simulink model "COVID_mod"  (Simulink 10.1)
settings: Solver=ode4  StartTime=0.0  StopTime=400  FixedStep=1  MaxStep=1e-2  RelTol=1e-3
values from neighbouring files (symbols this model uses):
  alpha = 1 / str2double( get( handles.tau_inc, 'String' ) )    [covid.m]
  beta = R * (gamma + Delta)    [covid.m]
  D_init = 0    [covid.m]
  delta = gamma    [covid.m]
  dOldRate = get( handles.ElderlyDeath, 'Value' )    [covid.m]
  dRate = 1 - get( handles.Recover, 'Value' )    [covid.m]
  E_init = 20 * I_init    [covid.m]
  gamma = 1/str2double( get( handles.tau_rec, 'String' ) )    [covid.m]
  Hi = 1 + tol    (= 1.05)    [covid.m]
  I_init = n    [covid.m]
  Lo = 1 - tol    (= 0.95)    [covid.m]
  N = str2double( get( handles.N, 'String' ) )    [covid.m]
  oldPop = get( handles.Elderly, 'Value' )    [covid.m]
  otherPop = 1 - oldPop    [covid.m]
  R_init = 0    [covid.m]
  S_init = N - I_init - E_init - D_init - R_init    [covid.m]
  sigma = get( hObject, 'Value' )    [covid.m]
  tau_sigmapost = str2double( get( handles.tau_sigmapost, 'String' ) )    [covid.m]
  tau_sigmapre = str2double( get( handles.tau_sigmapre, 'String' ) )    [covid.m]
  tau_xi = str2double( get( handles.tau_xi, 'String' ) )    [covid.m]
  xi = get( handles.Resusceptible, 'Value' ) / 100    [covid.m]
libraries: simulink x3
settings Model: Creator=markng  LastModifiedBy=markng
settings DataIOCC: SaveFormat=Dataset  ReturnWorkspaceOutputs=on  OutputSaveName=out
settings DebuggingCC: AlgebraicLoopMsg=none  ArtificialAlgebraicLoopMsg=none  UnderspecifiedInitializationDetection=Simplified  MergeDetectMultiDrivingBlocksExec=error  SFUnexpectedBacktrackingDiag=error  SFNoUnconditionalDefaultTransitionDiag=error
settings HardwareCC: ProdBitPerPointer=64  ProdLargestAtomicFloat=Float  ProdIntDivRoundTo=Zero  ProdEndianess=LittleEndian  ProdHWDeviceType=Specified
settings ModelReferenceCC: PropagateSignalLabelsOutOfModel=on
settings SFSimCC: SimUseLocalCustomCode=on
settings RTWCC: RTWUseLocalCustomCode=on
settings GRTTargetCC: TargetLangStandard=C99 (ISO)  CombineOutputUpdateFcns=on  GRTInterface=off
settings ConfigComp: CovMetricSettings=dwe  CovHtmlReporting=off  CovSaveCumulativeToWorkspaceVar=off  CovSaveSingleToWorkspaceVar=off  CovExternalEMLEnable=on

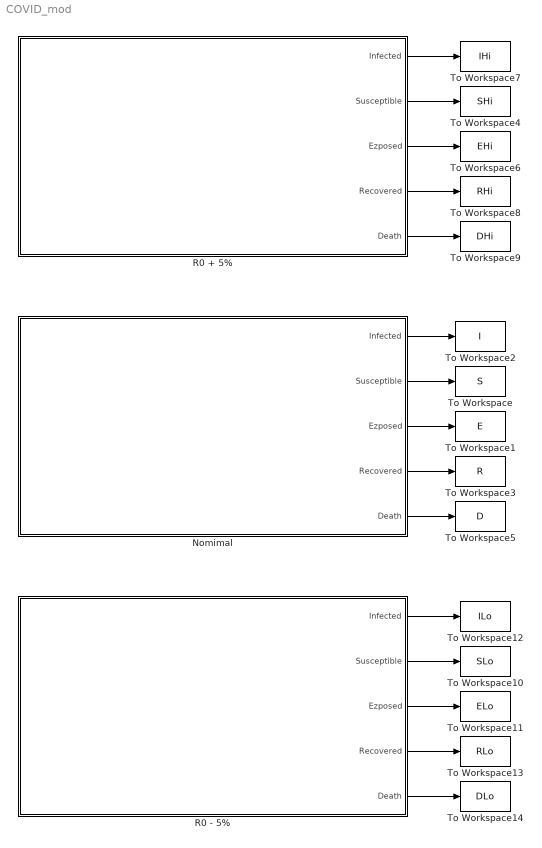
== system COVID_mod ==
  "Nomimal " : Subsystem
  R0 + 5% : Subsystem
  R0 - 5% : Subsystem
  To Workspace : ToWorkspace  VariableName=S  SaveFormat=Timeseries  SampleTime=-1
  To Workspace1 : ToWorkspace  VariableName=E  SaveFormat=Timeseries  SampleTime=-1
  To Workspace10 : ToWorkspace  VariableName=SLo  SaveFormat=Timeseries  SampleTime=-1
  To Workspace11 : ToWorkspace  VariableName=ELo  SaveFormat=Timeseries  SampleTime=-1
  To Workspace12 : ToWorkspace  VariableName=ILo  SaveFormat=Timeseries  SampleTime=-1
  To Workspace13 : ToWorkspace  VariableName=RLo  SaveFormat=Timeseries  SampleTime=-1
  To Workspace14 : ToWorkspace  VariableName=DLo  SaveFormat=Timeseries  SampleTime=-1
  To Workspace2 : ToWorkspace  VariableName=I  SaveFormat=Timeseries  SampleTime=-1
  To Workspace3 : ToWorkspace  VariableName=R  SaveFormat=Timeseries  SampleTime=-1
  To Workspace4 : ToWorkspace  VariableName=SHi  SaveFormat=Timeseries  SampleTime=-1
  To Workspace5 : ToWorkspace  VariableName=D  SaveFormat=Timeseries  SampleTime=-1
  To Workspace6 : ToWorkspace  VariableName=EHi  SaveFormat=Timeseries  SampleTime=-1
  To Workspace7 : ToWorkspace  VariableName=IHi  SaveFormat=Timeseries  SampleTime=-1
  To Workspace8 : ToWorkspace  VariableName=RHi  SaveFormat=Timeseries  SampleTime=-1
  To Workspace9 : ToWorkspace  VariableName=DHi  SaveFormat=Timeseries  SampleTime=-1
  wires:
  "Nomimal "/1(Infected) -> To Workspace2/1
  "Nomimal "/2(Susceptible) -> To Workspace/1
  "Nomimal "/3(Ezposed) -> To Workspace1/1
  "Nomimal "/4(Recovered) -> To Workspace3/1
  "Nomimal "/5(Death) -> To Workspace5/1
  R0 + 5%/2(Susceptible) -> To Workspace4/1
  R0 + 5%/4(Recovered) -> To Workspace8/1
  R0 + 5%/1(Infected) -> To Workspace7/1
  R0 + 5%/3(Ezposed) -> To Workspace6/1
  R0 + 5%/5(Death) -> To Workspace9/1
  R0 - 5%/2(Susceptible) -> To Workspace10/1
  R0 - 5%/4(Recovered) -> To Workspace13/1
  R0 - 5%/1(Infected) -> To Workspace12/1
  R0 - 5%/3(Ezposed) -> To Workspace11/1
  R0 - 5%/5(Death) -> To Workspace14/1

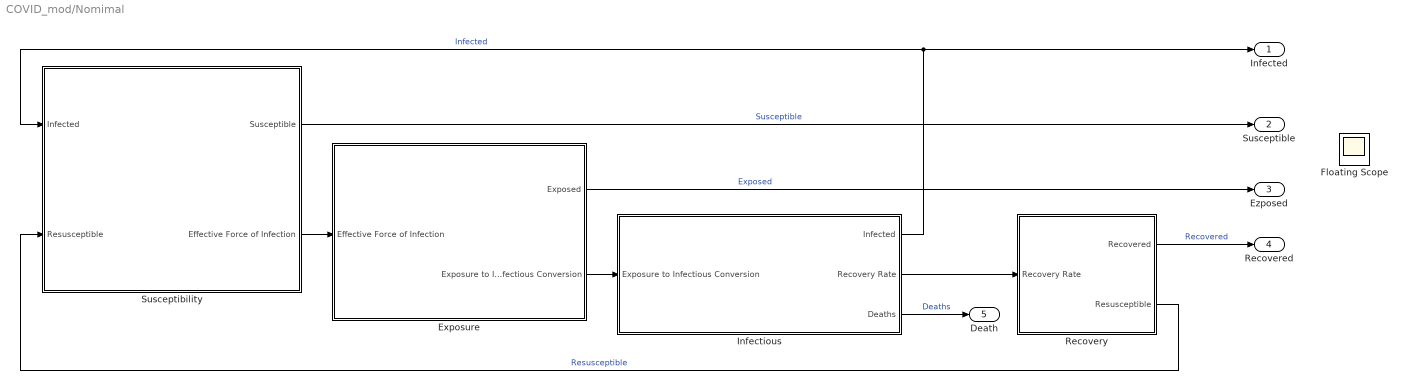
== system COVID_mod/Nomimal  ==
  Exposure : Subsystem
  Floating Scope : Scope
      settings: Floating=on
  Infectious : Subsystem
  Recovery : Subsystem
  Susceptibility : Subsystem
  Infected : Outport
  Susceptible : Outport  Port=2
  Ezposed : Outport  Port=3
  Recovered : Outport  Port=4
  Death : Outport  Port=5
  wires:
  Recovery/2(Resusceptible) -> Susceptibility/2(Resusceptible)  "Resusceptible"
  Susceptibility/1(Susceptible) -> Susceptible/1  "Susceptible"
  Exposure/2("Exposure to Infectious Conversion ") -> Infectious/1("Exposure to Infectious Conversion ")
  Susceptibility/2(Effective Force of Infection) -> Exposure/1(Effective Force of Infection)
  Exposure/1(Exposed) -> Ezposed/1  "Exposed"
  Infectious/1(Infected) -> Infected/1, Susceptibility/1(Infected)  "Infected"
  Recovery/1(Recovered) -> Recovered/1  "Recovered"
  Infectious/2(Recovery Rate) -> Recovery/1(Recovery Rate)
  Infectious/3(Deaths) -> Death/1  "Deaths"

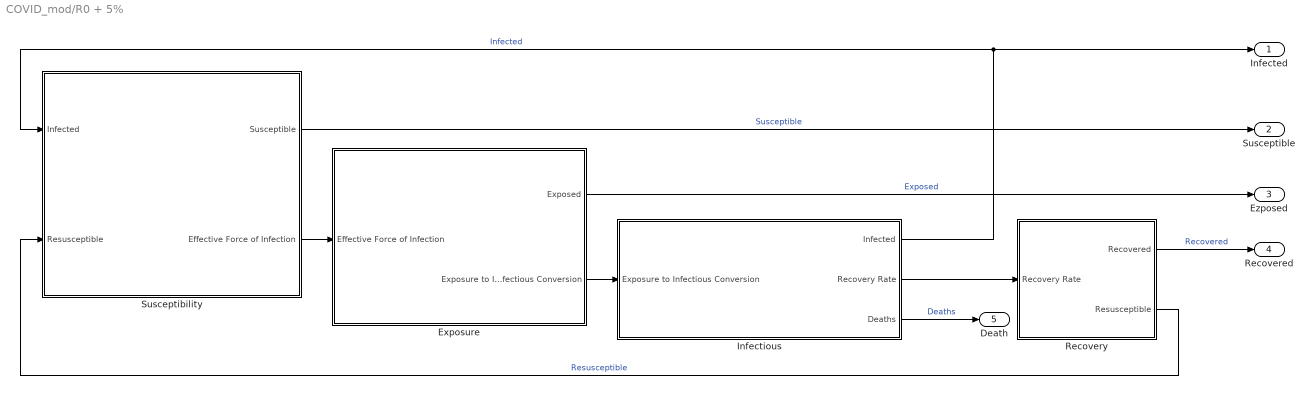
== system COVID_mod/R0 + 5% ==
  Exposure : Subsystem
  Infectious : Subsystem
  Recovery : Subsystem
  Susceptibility : Subsystem
  Infected : Outport
  Susceptible : Outport  Port=2
  Ezposed : Outport  Port=3
  Recovered : Outport  Port=4
  Death : Outport  Port=5
  wires:
  Recovery/2(Resusceptible) -> Susceptibility/2(Resusceptible)  "Resusceptible"
  Exposure/1(Exposed) -> Ezposed/1  "Exposed"
  Susceptibility/1(Susceptible) -> Susceptible/1  "Susceptible"
  Recovery/1(Recovered) -> Recovered/1  "Recovered"
  Infectious/1(Infected) -> Susceptibility/1(Infected), Infected/1  "Infected"
  Infectious/2(Recovery Rate) -> Recovery/1(Recovery Rate)
  Susceptibility/2(Effective Force of Infection) -> Exposure/1(Effective Force of Infection)
  Exposure/2("Exposure to Infectious Conversion ") -> Infectious/1("Exposure to Infectious Conversion ")
  Infectious/3(Deaths) -> Death/1  "Deaths"

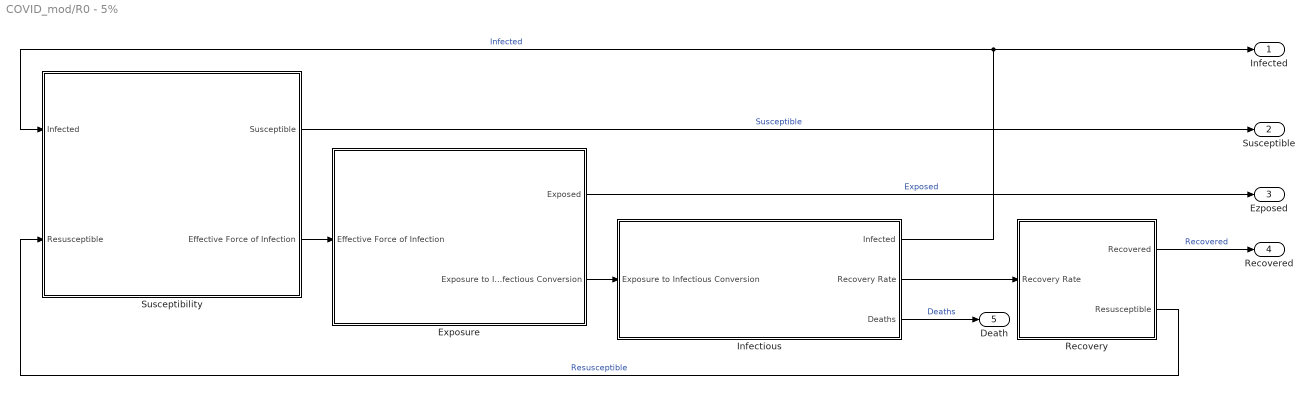
== system COVID_mod/R0 - 5% ==
  Exposure : Subsystem
  Infectious : Subsystem
  Recovery : Subsystem
  Susceptibility : Subsystem
  Infected : Outport
  Susceptible : Outport  Port=2
  Ezposed : Outport  Port=3
  Recovered : Outport  Port=4
  Death : Outport  Port=5
  wires:
  Recovery/2(Resusceptible) -> Susceptibility/2(Resusceptible)  "Resusceptible"
  Exposure/1(Exposed) -> Ezposed/1  "Exposed"
  Susceptibility/1(Susceptible) -> Susceptible/1  "Susceptible"
  Recovery/1(Recovered) -> Recovered/1  "Recovered"
  Infectious/1(Infected) -> Susceptibility/1(Infected), Infected/1  "Infected"
  Infectious/2(Recovery Rate) -> Recovery/1(Recovery Rate)
  Susceptibility/2(Effective Force of Infection) -> Exposure/1(Effective Force of Infection)
  Exposure/2("Exposure to Infectious Conversion ") -> Infectious/1("Exposure to Infectious Conversion ")
  Infectious/3(Deaths) -> Death/1  "Deaths"

== system COVID_mod/Nomimal /Exposure ==
  Effective Force of Infection : Inport
  Gain2 : Gain  Gain=alpha
  Integrator1 : Integrator  InitialCondition=E_init
  Sum1 : Sum  Inputs=|+-
  Exposed : Outport
  "Exposure to Infectious Conversion " : Outport  Port=2
  wires:
  Integrator1/1 -> Exposed/1, Gain2/1  "E"
  Sum1/1 -> Integrator1/1
  Effective Force of Infection/1 -> Sum1/1
  Gain2/1 -> Sum1/2, "Exposure to Infectious Conversion "/1

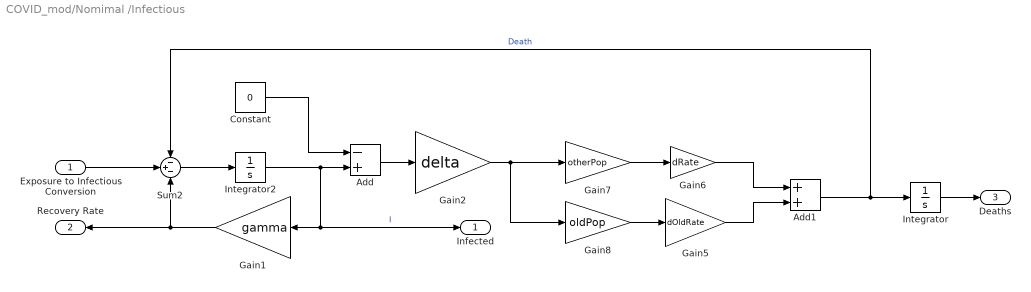
== system COVID_mod/Nomimal /Infectious ==
  "Exposure to Infectious Conversion " : Inport
  Add : Sum  Inputs=-+
  Add1 : Sum
  Constant : Constant  Value=0
  Gain1 : Gain  Gain=gamma
  Gain2 : Gain  Gain=delta
  Gain5 : Gain  Gain=dOldRate
  Gain6 : Gain  Gain=dRate
  Gain7 : Gain  Gain=otherPop
  Gain8 : Gain  Gain=oldPop
  Integrator : Integrator  InitialCondition=D_init
  Integrator2 : Integrator  InitialCondition=I_init
  Sum2 : Sum  Inputs=-+-
  Infected : Outport
  Recovery Rate : Outport  Port=2
  Deaths : Outport  Port=3
  wires:
  Sum2/1 -> Integrator2/1
  "Exposure to Infectious Conversion "/1 -> Sum2/2
  Gain1/1 -> Sum2/3, Recovery Rate/1
  Gain7/1 -> Gain6/1
  Gain8/1 -> Gain5/1
  Add1/1 -> Integrator/1, Sum2/1  "Death"
  Integrator2/1 -> Add/2, Infected/1, Gain1/1  "I"
  Gain6/1 -> Add1/1
  Integrator/1 -> Deaths/1
  Gain5/1 -> Add1/2
  Constant/1 -> Add/1
  Add/1 -> Gain2/1
  Gain2/1 -> Gain8/1, Gain7/1

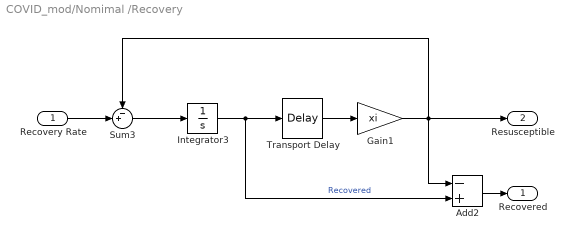
== system COVID_mod/Nomimal /Recovery ==
  Recovery Rate : Inport
  Add2 : Sum  Inputs=-+
  Gain1 : Gain  Gain=xi
  Integrator3 : Integrator  InitialCondition=R_init
  Sum3 : Sum  Inputs=-+|
  Transport Delay : TransportDelay  DelayTime=tau_xi
  Recovered : Outport
  Resusceptible : Outport  Port=2
  wires:
  Recovery Rate/1 -> Sum3/2
  Integrator3/1 -> Transport Delay/1, Add2/2  "Recovered"
  Sum3/1 -> Integrator3/1
  Add2/1 -> Recovered/1
  Gain1/1 -> Resusceptible/1, Sum3/1, Add2/1
  Transport Delay/1 -> Gain1/1

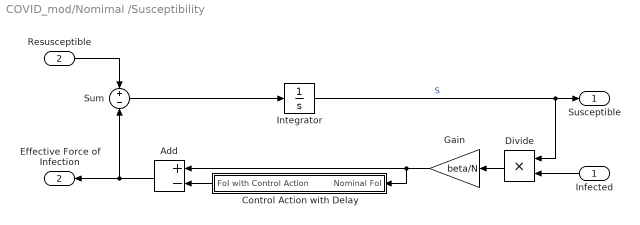
== system COVID_mod/Nomimal /Susceptibility ==
  Infected : Inport
  Resusceptible : Inport  Port=2
  Add : Sum  Inputs=+-
  Control Action with Delay : Subsystem
  Divide : Product  Inputs=**
  Gain : Gain  Gain=beta/N
  Integrator : Integrator  InitialCondition=S_init
  Sum : Sum  Inputs=+-
  Susceptible : Outport
  Effective Force of Infection : Outport  Port=2
  wires:
  Infected/1 -> Divide/2
  Divide/1 -> Gain/1
  Control Action with Delay/1(FoI with Control Action) -> Add/2
  Gain/1 -> Control Action with Delay/1(Nominal FoI), Add/1
  Integrator/1 -> Susceptible/1, Divide/1  "S"
  Add/1 -> Sum/2, Effective Force of Infection/1
  Resusceptible/1 -> Sum/1
  Sum/1 -> Integrator/1

== system COVID_mod/R0 + 5%/Exposure ==
  Effective Force of Infection : Inport
  Gain2 : Gain  Gain=alpha
  Integrator1 : Integrator  InitialCondition=E_init
  Sum1 : Sum  Inputs=|+-
  Exposed : Outport
  "Exposure to Infectious Conversion " : Outport  Port=2
  wires:
  Integrator1/1 -> Exposed/1, Gain2/1  "E"
  Sum1/1 -> Integrator1/1
  Effective Force of Infection/1 -> Sum1/1
  Gain2/1 -> Sum1/2, "Exposure to Infectious Conversion "/1

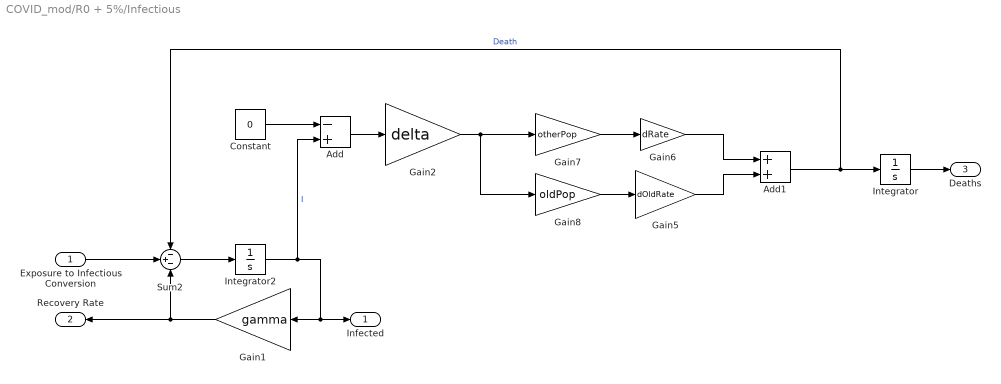
== system COVID_mod/R0 + 5%/Infectious ==
  "Exposure to Infectious Conversion " : Inport
  Add : Sum  Inputs=-+
  Add1 : Sum
  Constant : Constant  Value=0
  Gain1 : Gain  Gain=gamma
  Gain2 : Gain  Gain=delta
  Gain5 : Gain  Gain=dOldRate
  Gain6 : Gain  Gain=dRate
  Gain7 : Gain  Gain=otherPop
  Gain8 : Gain  Gain=oldPop
  Integrator : Integrator  InitialCondition=D_init
  Integrator2 : Integrator  InitialCondition=I_init
  Sum2 : Sum  Inputs=-+-
  Infected : Outport
  Recovery Rate : Outport  Port=2
  Deaths : Outport  Port=3
  wires:
  Sum2/1 -> Integrator2/1
  "Exposure to Infectious Conversion "/1 -> Sum2/2
  Gain1/1 -> Sum2/3, Recovery Rate/1
  Gain7/1 -> Gain6/1
  Gain8/1 -> Gain5/1
  Add1/1 -> Integrator/1, Sum2/1  "Death"
  Integrator2/1 -> Add/2, Infected/1, Gain1/1  "I"
  Gain6/1 -> Add1/1
  Integrator/1 -> Deaths/1
  Gain5/1 -> Add1/2
  Constant/1 -> Add/1
  Add/1 -> Gain2/1
  Gain2/1 -> Gain8/1, Gain7/1

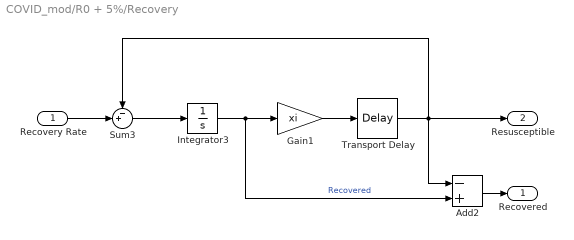
== system COVID_mod/R0 + 5%/Recovery ==
  Recovery Rate : Inport
  Add2 : Sum  Inputs=-+
  Gain1 : Gain  Gain=xi
  Integrator3 : Integrator  InitialCondition=R_init
  Sum3 : Sum  Inputs=-+|
  Transport Delay : TransportDelay  DelayTime=tau_xi
  Recovered : Outport
  Resusceptible : Outport  Port=2
  wires:
  Recovery Rate/1 -> Sum3/2
  Integrator3/1 -> Gain1/1, Add2/2  "Recovered"
  Sum3/1 -> Integrator3/1
  Add2/1 -> Recovered/1
  Gain1/1 -> Transport Delay/1
  Transport Delay/1 -> Sum3/1, Add2/1, Resusceptible/1

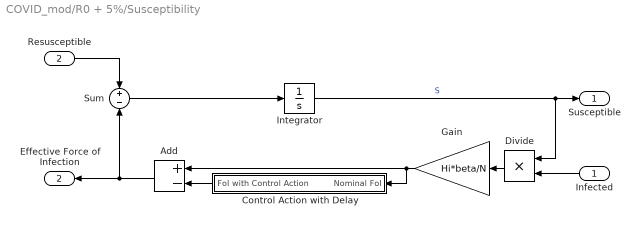
== system COVID_mod/R0 + 5%/Susceptibility ==
  Infected : Inport
  Resusceptible : Inport  Port=2
  Add : Sum  Inputs=+-
  Control Action with Delay : Subsystem
  Divide : Product  Inputs=**
  Gain : Gain  Gain=Hi*beta/N
  Integrator : Integrator  InitialCondition=S_init
  Sum : Sum  Inputs=+-
  Susceptible : Outport
  Effective Force of Infection : Outport  Port=2
  wires:
  Infected/1 -> Divide/2
  Divide/1 -> Gain/1
  Control Action with Delay/1(FoI with Control Action) -> Add/2
  Gain/1 -> Control Action with Delay/1(Nominal FoI), Add/1
  Integrator/1 -> Susceptible/1, Divide/1  "S"
  Add/1 -> Sum/2, Effective Force of Infection/1
  Resusceptible/1 -> Sum/1
  Sum/1 -> Integrator/1

== system COVID_mod/R0 - 5%/Exposure ==
  Effective Force of Infection : Inport
  Gain2 : Gain  Gain=alpha
  Integrator1 : Integrator  InitialCondition=E_init
  Sum1 : Sum  Inputs=|+-
  Exposed : Outport
  "Exposure to Infectious Conversion " : Outport  Port=2
  wires:
  Integrator1/1 -> Exposed/1, Gain2/1  "E"
  Sum1/1 -> Integrator1/1
  Effective Force of Infection/1 -> Sum1/1
  Gain2/1 -> Sum1/2, "Exposure to Infectious Conversion "/1

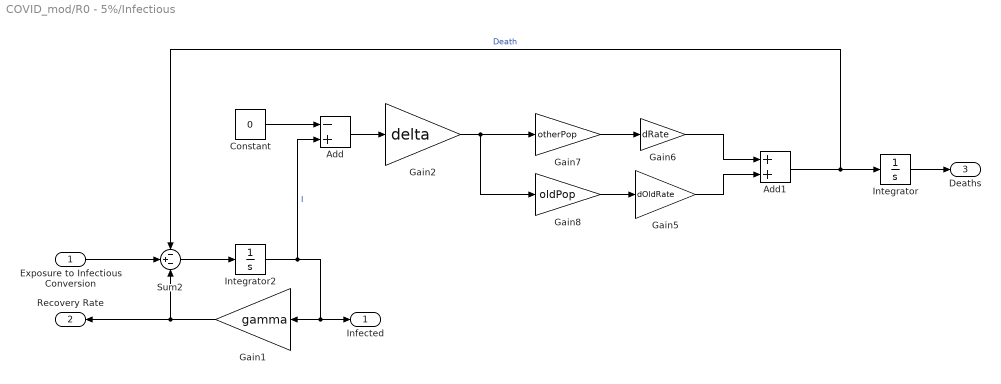
== system COVID_mod/R0 - 5%/Infectious ==
  "Exposure to Infectious Conversion " : Inport
  Add : Sum  Inputs=-+
  Add1 : Sum
  Constant : Constant  Value=0
  Gain1 : Gain  Gain=gamma
  Gain2 : Gain  Gain=delta
  Gain5 : Gain  Gain=dOldRate
  Gain6 : Gain  Gain=dRate
  Gain7 : Gain  Gain=otherPop
  Gain8 : Gain  Gain=oldPop
  Integrator : Integrator  InitialCondition=D_init
  Integrator2 : Integrator  InitialCondition=I_init
  Sum2 : Sum  Inputs=-+-
  Infected : Outport
  Recovery Rate : Outport  Port=2
  Deaths : Outport  Port=3
  wires:
  Sum2/1 -> Integrator2/1
  "Exposure to Infectious Conversion "/1 -> Sum2/2
  Gain1/1 -> Sum2/3, Recovery Rate/1
  Gain7/1 -> Gain6/1
  Gain8/1 -> Gain5/1
  Add1/1 -> Integrator/1, Sum2/1  "Death"
  Integrator2/1 -> Add/2, Infected/1, Gain1/1  "I"
  Gain6/1 -> Add1/1
  Integrator/1 -> Deaths/1
  Gain5/1 -> Add1/2
  Constant/1 -> Add/1
  Add/1 -> Gain2/1
  Gain2/1 -> Gain8/1, Gain7/1

== system COVID_mod/R0 - 5%/Recovery ==
  Recovery Rate : Inport
  Add2 : Sum  Inputs=-+
  Gain1 : Gain  Gain=xi
  Integrator3 : Integrator  InitialCondition=R_init
  Sum3 : Sum  Inputs=-+|
  Transport Delay : TransportDelay  DelayTime=tau_xi
  Recovered : Outport
  Resusceptible : Outport  Port=2
  wires:
  Recovery Rate/1 -> Sum3/2
  Integrator3/1 -> Gain1/1, Add2/2  "Recovered"
  Sum3/1 -> Integrator3/1
  Add2/1 -> Recovered/1
  Gain1/1 -> Transport Delay/1
  Transport Delay/1 -> Sum3/1, Add2/1, Resusceptible/1

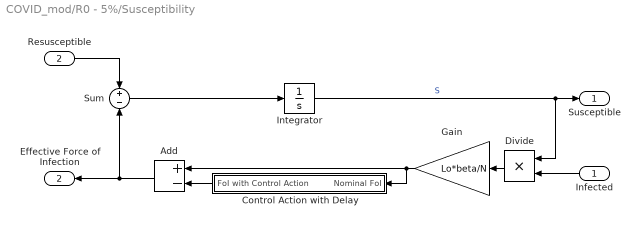
== system COVID_mod/R0 - 5%/Susceptibility ==
  Infected : Inport
  Resusceptible : Inport  Port=2
  Add : Sum  Inputs=+-
  Control Action with Delay : Subsystem
  Divide : Product  Inputs=**
  Gain : Gain  Gain=Lo*beta/N
  Integrator : Integrator  InitialCondition=S_init
  Sum : Sum  Inputs=+-
  Susceptible : Outport
  Effective Force of Infection : Outport  Port=2
  wires:
  Infected/1 -> Divide/2
  Divide/1 -> Gain/1
  Control Action with Delay/1(FoI with Control Action) -> Add/2
  Gain/1 -> Add/1, Control Action with Delay/1(Nominal FoI)
  Integrator/1 -> Susceptible/1, Divide/1  "S"
  Add/1 -> Sum/2, Effective Force of Infection/1
  Resusceptible/1 -> Sum/1
  Sum/1 -> Integrator/1

== system COVID_mod/Nomimal /Susceptibility/Control Action with Delay ==
  Nominal FoI : Inport
  Clock : Clock
  Compare To Constant : simulink/Logic and Bit Operations/Compare To Constant  relop=>=  const=tau_sigmapre + tau_sigmapost  OutDataTypeStr=boolean
  Divide : Product  Inputs=**
  Gain1 : Gain  Gain=sigma
  FoI with Control Action : Outport
  wires:
  Nominal FoI/1 -> Divide/2
  Divide/1 -> Gain1/1
  Gain1/1 -> FoI with Control Action/1
  Clock/1 -> Compare To Constant/1
  Compare To Constant/1 -> Divide/1

== system COVID_mod/R0 + 5%/Susceptibility/Control Action with Delay ==
  Nominal FoI : Inport
  Clock : Clock
  Compare To Constant : simulink/Logic and Bit Operations/Compare To Constant  relop=>=  const=tau_sigmapre + tau_sigmapost  OutDataTypeStr=boolean
  Divide : Product  Inputs=**
  Gain1 : Gain  Gain=sigma
  FoI with Control Action : Outport
  wires:
  Nominal FoI/1 -> Divide/2
  Divide/1 -> Gain1/1
  Gain1/1 -> FoI with Control Action/1
  Clock/1 -> Compare To Constant/1
  Compare To Constant/1 -> Divide/1

== system COVID_mod/R0 - 5%/Susceptibility/Control Action with Delay ==
  Nominal FoI : Inport
  Clock : Clock
  Compare To Constant : simulink/Logic and Bit Operations/Compare To Constant  relop=>=  const=tau_sigmapre + tau_sigmapost  OutDataTypeStr=boolean
  Divide : Product  Inputs=**
  Gain1 : Gain  Gain=sigma
  FoI with Control Action : Outport
  wires:
  Nominal FoI/1 -> Divide/2
  Divide/1 -> Gain1/1
  Gain1/1 -> FoI with Control Action/1
  Clock/1 -> Compare To Constant/1
  Compare To Constant/1 -> Divide/1
